simulink subsystem "Model_gravity"  (R2023a)
settings: Solver=VariableStepAuto  StartTime=0.0  StopTime=10.0  RelTol=1e-3
undefined symbols (not defined in the file): param
settings Model: Creator=raduserseniuc  LastModifiedBy=raduserseniuc

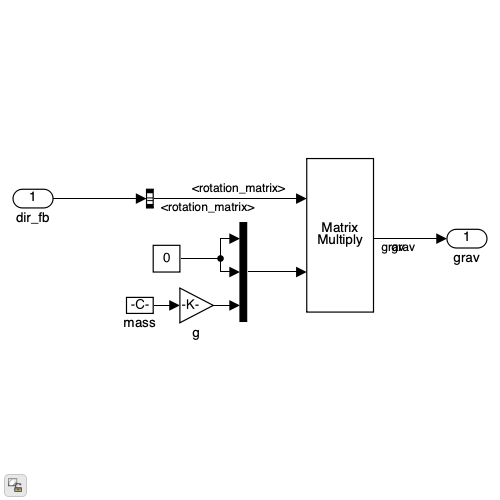
[thumbnail: Simulink's stored preview of the top-level diagram]
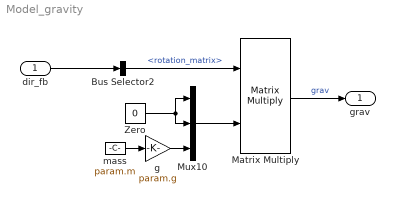
== system Model_gravity ==
  dir_fb : Inport
  Bus Selector2 : BusSelector  OutputSignals=rotation_matrix
  Matrix Multiply : Product  Inputs=**  Multiplication=Matrix(*)
  Mux10 : Mux  Inputs=3
  Zero : Constant  Value=0  OutDataTypeStr=Inherit: Inherit via back propagation
  g : Gain  Gain=param.g
  mass : Constant  Value=param.m
  grav : Outport
  wires:
  Mux10/1 -> Matrix Multiply/2
  Matrix Multiply/1 -> grav/1  "grav"
  Bus Selector2/1 -> Matrix Multiply/1  "<rotation_matrix>"
  g/1 -> Mux10/3
  dir_fb/1 -> Bus Selector2/1
  Zero/1 -> Mux10/2, Mux10/1
  mass/1 -> g/1
